simulink model "coursework2model9"  (R2018b)
settings: Solver=FixedStepAuto  StartTime=0.0  StopTime=60  FixedStep=Ts  RelTol=1e-3
InitFcn:
  | paramsCW2_v8
values from neighbouring files (symbols this model uses):
  C = [1 0 0 0;0 1 0 0]    [paramsCW2_v8.m]
  K = lqr([0 1 0 0 0;[0;0;0;0] A],[0;B],[1 0 0 0 0; [0;0;0;0] Q],R)    [paramsCW2_v8.m]
  n = 5    [paramsCW2_v8.m]
undefined symbols (not defined in the file or in its folder): sso
settings Model: Creator=jakubkryczka  LastModifiedBy=jakubkryczka
settings DebuggingCC: LibraryContextMissingDiagnostic=none
settings SFSimCC: SimUseLocalCustomCode=off
settings RTWCC: RTWUseLocalCustomCode=off

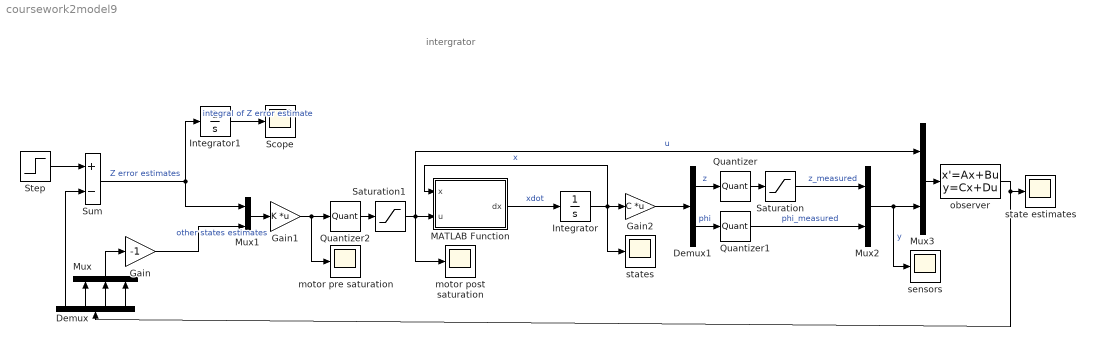
== system coursework2model9 ==
  note: intergrator
  Demux : Demux
  Demux1 : Demux  Outputs=2
  Gain : Gain  Gain=-1
  Gain1 : Gain  Gain=K  Multiplication=Matrix(K*u)
  Gain2 : Gain  Gain=C  Multiplication=Matrix(K*u)
  Integrator : Integrator  InitialCondition=[0;0;0;0]
  Integrator1 : Integrator
  MATLAB Function : MATLAB Function  TreatAsAtomicUnit=on
  Mux : Mux  Inputs=3
  Mux1 : Mux  Inputs=2
  Mux2 : Mux  Inputs=2
  Mux3 : Mux  Inputs=2
  Quantizer : Quantizer  QuantizationInterval=0.001
  Quantizer1 : Quantizer  QuantizationInterval=pi/(180*n)
  Quantizer2 : Quantizer  QuantizationInterval=14/100
  Saturation : Saturate
  Saturation1 : Saturate  UpperLimit=14  LowerLimit=-14
  Scope : Scope
  Step : Step  After=0.2  SampleTime=0
  Sum : Sum  Inputs=+-
  motor post saturation : Scope
  motor pre saturation : Scope
  observer : StateSpace  A=sso.A  B=sso.B  C=eye(4)  D=zeros(4,3)  InitialCondition=[0;0;0;0]
  sensors : Scope
  state estimates : Scope
  states : Scope
  wires:
  Sum/1 -> Mux1/1, Integrator1/1  "Z error estimates"
  Step/1 -> Sum/1
  Demux/2 -> Mux/1
  Demux/3 -> Mux/2
  Demux/4 -> Mux/3
  Mux/1 -> Gain/1
  Demux/1 -> Sum/2
  Gain/1 -> Mux1/2  "other states estimates"
  Saturation1/1 -> MATLAB Function/2(u), Mux3/1, motor post saturation/1  "u"
  Demux1/1 -> Quantizer/1  "z"
  Demux1/2 -> Quantizer1/1  "phi"
  Quantizer/1 -> Saturation/1
  Mux2/1 -> Mux3/2, sensors/1  "y"
  Saturation/1 -> Mux2/1  "z_measured"
  Quantizer1/1 -> Mux2/2  "phi_measured"
  Quantizer2/1 -> Saturation1/1
  Gain2/1 -> Demux1/1
  Mux3/1 -> observer/1
  observer/1 -> Demux/1, state estimates/1
  MATLAB Function/1(dx) -> Integrator/1  "xdot"
  Integrator/1 -> states/1, Gain2/1, MATLAB Function/1(x)  "x"
  Gain1/1 -> motor pre saturation/1, Quantizer2/1
  Integrator1/1 -> Scope/1  "integral of Z error estimate"
  Mux1/1 -> Gain1/1

== matlab function coursework2model9/MATLAB Function ==
  data: x input; u input; dx output
function dx = fcn(x,u)
beta = 0.01;
alpha = 0.01;
J = 0.2;
g = 9.81;
m = 0.05;
n = 5;

b = beta*n^2;
k = alpha*n;

dx = [x(3);
    x(4);
    (x(1)*((x(4))^2)-(g*sin(x(2))))/1.8;
    ((k*u)-(2*m*x(1)*x(3)*x(4))-(m*g*x(1)*cos(x(2)))-(b*x(4)))/(J+(m*((x(1))^2)))];

end
